simulink model "Automaton"  (R2015a)
settings: Solver=ode45  StartTime=0.0  StopTime=10.0  RelTol=1e-3
settings Model: Creator=DieHenz  LastModifiedBy=DieHenz

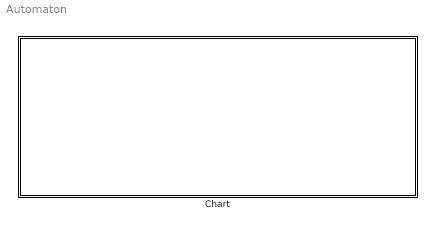
== system Automaton ==
  Chart : Stateflow chart  TreatAsAtomicUnit=on

== stateflow chart Automaton/Chart ==
  state Robot
    state Rotation
      entry: kp=0.1;
      kg=0.001;
    state Line_Follower
      entry: kp=0.001;
      kg=0.1;
    state Idle
      entry: kp=0;
      Kg=0;
    (default) -> Rotation
    Rotation -> Line_Follower : theta_error < 1°
    Idle -> Rotation : [sqrt((xg-x)^2+(yg-y)^2) > 10]
    Line_Follower -> Idle : [sqrt((xg-x)^2+(yg-y)^2) < 5]
  state X_goal [group]
  state Y_goal [group]
  X_goal -> Robot
  Y_goal -> Robot
